simulink model "questao2"  (R2023a)
settings: Solver=VariableStepAuto  StartTime=0.0  StopTime=100  RelTol=1e-3
values from neighbouring files (symbols this model uses):
  B = 0.1    [Trab1_real.m]    (also in questao5.m)
  K = 1/3    (= 0.333333333333)    [Trab1_real.m]    (also in questao5.m)
  L = 0.5    [Trab1_real.m]    (also in questao5.m)
  R = 10    [Trab1_real.m]    (also in questao5.m)
settings Model: Creator=pedro  LastModifiedBy=pedro

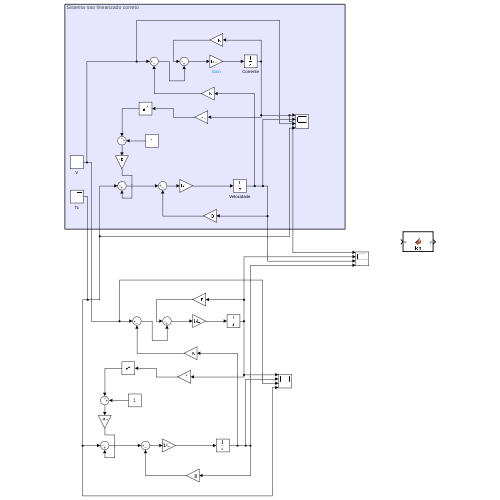
[thumbnail: Simulink's stored preview of the top-level diagram]
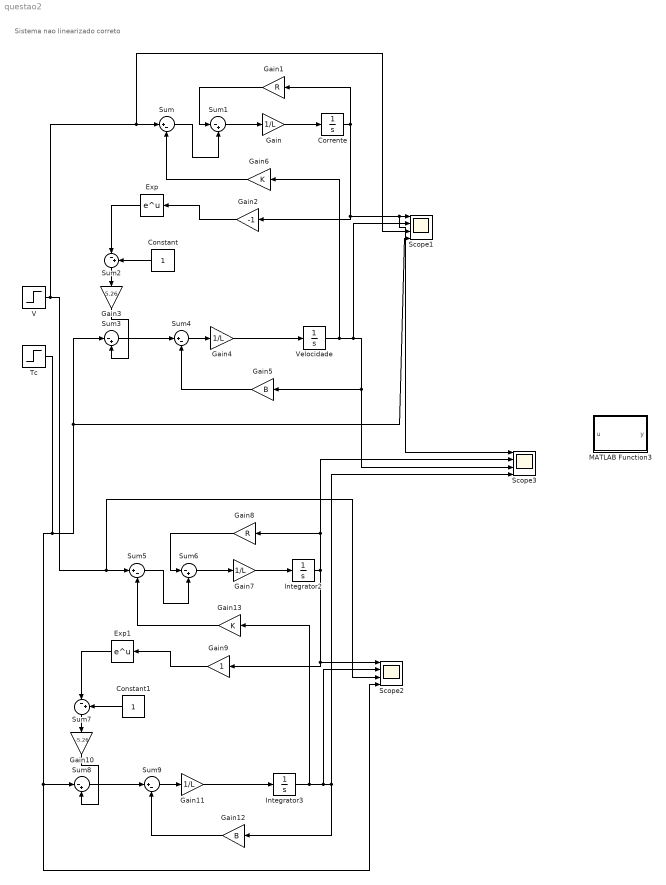
== system questao2 ==
  note: Sistema nao linearizado correto
  Constant : Constant
  Constant1 : Constant
  Corrente : Integrator
  Exp : Math
  Exp1 : Math
  Gain{,4,7,11} (4 alike) : Gain  Gain=1/L
  Gain1 : Gain  Gain=R
  Gain10 : Gain  Gain=-5.26
  Gain12 : Gain  Gain=B
  Gain13 : Gain  Gain=K
  Gain2 : Gain  Gain=-1
  Gain3 : Gain  Gain=5.26
  Gain5 : Gain  Gain=B
  Gain6 : Gain  Gain=K
  Gain8 : Gain  Gain=R
  Gain9 : Gain
  Integrator2 : Integrator
  Integrator3 : Integrator
  MATLAB Function3 : MATLAB Function  TreatAsAtomicUnit=on
  Scope1 : Scope  NumInputPorts=4
  Scope2 : Scope  NumInputPorts=4
  Scope3 : Scope  NumInputPorts=4
  Sum{,4..5,9} (4 alike) : Sum  Inputs=|+-
  Sum{1..3,6..8} (6 alike) : Sum  Inputs=|-+
  Tc : Step  Time=10  After=2  SampleTime=0
  V : Step  Time=10  After=9.16  SampleTime=0
  Velocidade : Integrator
  wires:
  V/1 -> Scope1/3, Sum/1, Scope2/3, Sum5/1
  Sum1/1 -> Gain/1
  Gain/1 -> Corrente/1
  Corrente/1 -> Gain2/1, Scope3/1, Scope1/1, Gain1/1
  Gain2/1 -> Exp/1
  Gain1/1 -> Sum1/1
  Sum/1 -> Sum1/2
  Exp/1 -> Sum2/1
  Constant/1 -> Sum2/2
  Sum2/1 -> Gain3/1
  Tc/1 -> Scope2/4, Sum8/1, Sum3/1, Scope1/4
  Sum3/1 -> Sum4/1
  Gain3/1 -> Sum3/2
  Sum4/1 -> Gain4/1
  Gain4/1 -> Velocidade/1
  Velocidade/1 -> Scope1/2, Scope3/3, Gain5/1, Gain6/1
  Gain5/1 -> Sum4/2
  Gain6/1 -> Sum/2
  Gain9/1 -> Exp1/1
  Sum5/1 -> Sum6/2
  Gain7/1 -> Integrator2/1
  Exp1/1 -> Sum7/1
  Constant1/1 -> Sum7/2
  Sum6/1 -> Gain7/1
  Gain10/1 -> Sum8/2
  Gain13/1 -> Sum5/2
  Sum8/1 -> Sum9/1
  Gain12/1 -> Sum9/2
  Sum9/1 -> Gain11/1
  Sum7/1 -> Gain10/1
  Gain8/1 -> Sum6/1
  Integrator2/1 -> Gain9/1, Scope2/1, Scope3/2, Gain8/1
  Gain11/1 -> Integrator3/1
  Integrator3/1 -> Scope2/2, Scope3/4, Gain12/1, Gain13/1

== matlab function questao2/MATLAB Function3 ==
  data: u input; y output
function y = fcn(u)

y = u;
